simulink model "a"  (R2012b)
settings: Solver=ode45  StartTime=0.0  StopTime=100  RelTol=1e-3
settings Model: Creator=ZhouHaoyu  LastModifiedBy=ZhouHaoyu

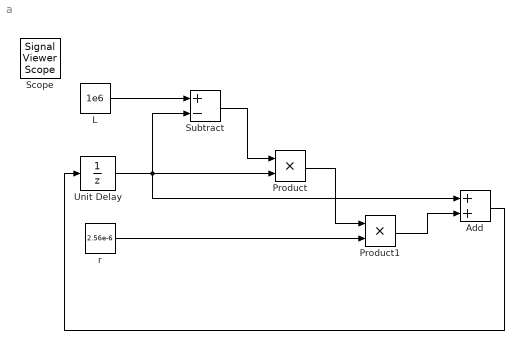
== system a ==
  Add : Sum
  L : Constant  Value=1e6
  Product : Product  RndMeth=Zero
  Product1 : Product  RndMeth=Zero
  Subtract : Sum  Inputs=+-
  Unit Delay : UnitDelay  InitialCondition=1e5
  r : Constant  Value=2.56e-6
  Scope : SignalViewerScope  IOType=viewer  RefreshTime=0.035000
  wires:
  L/1 -> Subtract/1
  Unit Delay/1 -> Subtract/2, Add/1, Product/2
  Subtract/1 -> Product/1
  r/1 -> Product1/2
  Product/1 -> Product1/1
  Product1/1 -> Add/2
  Add/1 -> Unit Delay/1
